simulink model "sistema_completo_discretizado_con_funciones"  (R2023b)
settings: Solver=VariableStepAuto  StartTime=0.0  StopTime=10.0  RelTol=1e-3
values from neighbouring files (symbols this model uses):
  alpha_Cu = 3.9e-3    (= 0.0039)    [controlador_foc_simulink.m]    (also in parametros_planta.m; params_subsistema_termico.m; sistema_completo_en_codigo.m)
  beq_nom = bm + bl_nom/r^2    (= 2.19444444444e-05)    [parametros_planta.m]    (also in params_subsistema_mecanico.m; sistema_completo_en_codigo.m)
  Cts = 0.818    [parametros_planta.m]    (also in params_subsistema_termico.m)
  Jeq_nom = Jm + Jl_nom/r^2    (= 1.97847222222e-05)    [params_subsistema_mecanico.m]    (also in sistema_completo_en_codigo.m)
  kg_eq_nom = g*kl_nom/r    (= 0.0204305208333)    [params_subsistema_mecanico.m]    (also in sistema_completo_en_codigo.m)
  L_d = 6.6e-3    (= 0.0066)    [controlador_foc_simulink.m]    (also in params_subsistema_electromagnetico.m; sistema_completo_en_codigo.m)
  L_l = 0.8e-3    (= 0.0008)    [controlador_foc_simulink.m]    (also in params_subsistema_electromagnetico.m; sistema_completo_en_codigo.m)
  L_q = 5.8e-3    (= 0.0058)    [controlador_foc_simulink.m]    (also in params_subsistema_electromagnetico.m; sistema_completo_en_codigo.m)
  lambda_m = 0.016    [controlador_foc_simulink.m]    (also in parametros_planta.m; params_subsistema_electromagnetico.m; sistema_completo_en_codigo.m)
  Pp = 3    [controlador_foc_simulink.m]    (also in parametros_planta.m; params_subsistema_electromagnetico.m; sistema_completo_en_codigo.m)
  r = 120.0    (= 120)    [controlador_foc_simulink.m]    (also in parametros_planta.m; params_subsistema_mecanico.m; sistema_completo_en_codigo.m)
  Rs_REF = 1.02    [controlador_foc_simulink.m]    (also in parametros_planta.m; params_subsistema_termico.m; sistema_completo_en_codigo.m)
  Rts_amb = 146.7    [parametros_planta.m]    (also in params_subsistema_termico.m)
  Tamb = Tamb_max    (= 40)    [parametros_planta.m]    (also in params_subsistema_termico.m; sistema_completo_en_codigo.m)
  Ts = interp_ts(Ts_ts,t)    [calcular_metricas_operacion.m]
  Ts_REF = 20.0    (= 20)    [controlador_foc_simulink.m]    (also in parametros_planta.m; params_subsistema_termico.m; sistema_completo_en_codigo.m)
undefined symbols (not defined in the file or in its folder): A_iabc, A_pos, A_T, A_v, B_iabc, B_pos, B_T, B_v, C_iabc, C_pos, C_T, C_v, D_iabc, D_pos, D_T, D_v
settings Model: Creator=Pc  LastModifiedBy=Pc

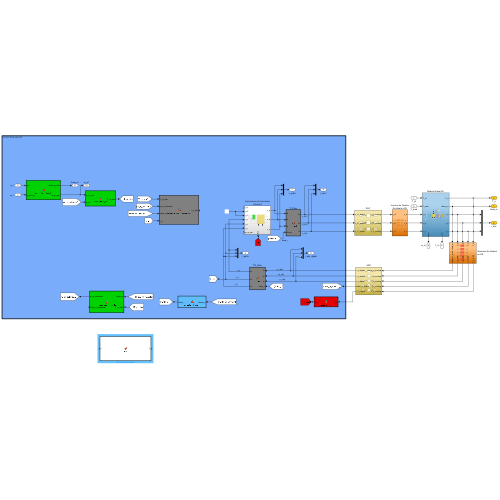
[thumbnail: Simulink's stored preview of the top-level diagram]
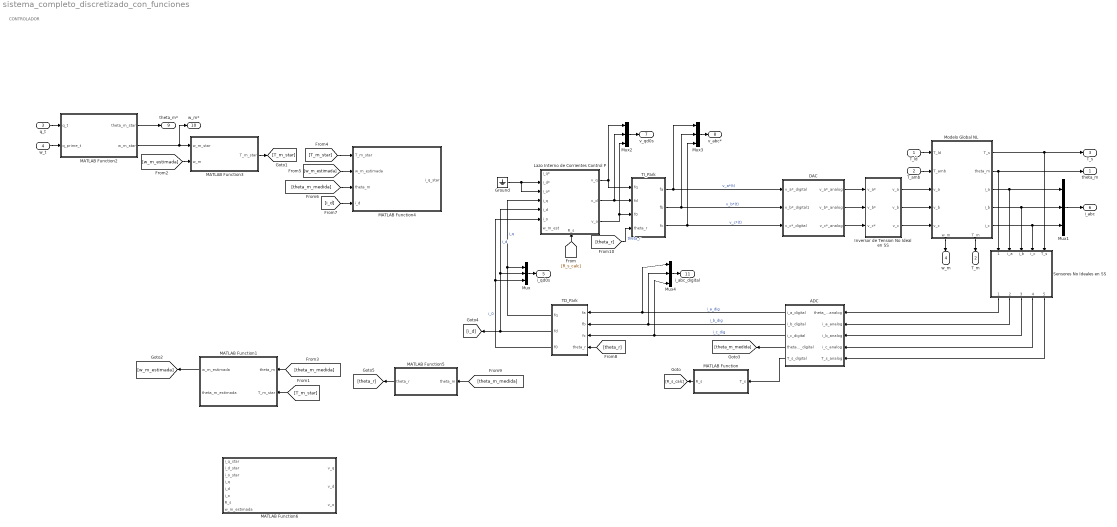
== system sistema_completo_discretizado_con_funciones ==
  note: CONTROLADOR
  T_ld : Inport
  T_amb : Inport  Port=2
  q_t : Inport  Port=3
  w_t : Inport  Port=4
  " ADC" : Subsystem
  DAC : Subsystem
  Ground : Ground
  Inversor de Tension No Ideal en SS : Subsystem
  Lazo Interno de Corrientes Control P : Subsystem
      settings: PortSchema="{\"entries\":[{\"content\":{\"sides\":[{\"content\":{\"connectorIds\":[\"In1\",\"In2\",\"In3\",\"In4\",\"In5\",\"In6\",\"In7\"]},\"type\":\"ConnectorPlacement.EquallySpacedRectSide\",\"uuid\":\"003130de-7086-42b2-88ab-1550be464119\"},{\"content\":{\"connectorIds\":[\"Out1\",\"Out2\",\"Out3\"],\"side\":\"RIGHT\"},\"type\":\"ConnectorPlacement.EquallySpacedRectSide\",\"uuid\":\"1ef26d10-ae91-4351-8dbc-50b579db1e66\"},{\"content\":{\"side\":\"TOP\"},\"type\":\"ConnectorPlacement.EquallySpacedRectSide\",\"uuid\":\"f8d5b360-b304-4c62-a3c0-e85b3671d199\"},{\"content\":{\"connectorIds\":[\"In8\"],\"side\":\"BOTTOM\"},\"type\":\"ConnectorPlacement.EquallySpacedRectSide\",\"uuid\":\"ca7bddea-434a-49b1-aeae-36f1f1b68346\"}]},\"type\":\"ConnectorPlacement.EquallySpacedConnector\",\"uuid\":\"97d0594b-d096-4b47-8675-ea576c5ffe32\"}],\"packageUris\":[\"http://schema.mathworks.com/mf0/Connector/R2020b\"],\"version\":\"1.0\"}"
  MATLAB Function : MATLAB Function  TreatAsAtomicUnit=on
  MATLAB Function1 : MATLAB Function  TreatAsAtomicUnit=on
  MATLAB Function2 : MATLAB Function  TreatAsAtomicUnit=on
  MATLAB Function3 : MATLAB Function  TreatAsAtomicUnit=on
  MATLAB Function4 : MATLAB Function  TreatAsAtomicUnit=on
  MATLAB Function5 : MATLAB Function  TreatAsAtomicUnit=on
  MATLAB Function6 : MATLAB Function  TreatAsAtomicUnit=on
  Modelo Global NL : Subsystem
      settings: PortSchema="{\"entries\":[{\"content\":{\"sides\":[{\"content\":{\"connectorIds\":[\"In1\",\"In2\",\"In3\",\"In4\",\"In5\"]},\"type\":\"ConnectorPlacement.EquallySpacedRectSide\",\"uuid\":\"386252be-5f39-4928-a151-52e681895a84\"},{\"content\":{\"connectorIds\":[\"Out1\",\"Out2\",\"Out3\",\"Out4\",\"Out5\"],\"side\":\"RIGHT\"},\"type\":\"ConnectorPlacement.EquallySpacedRectSide\",\"uuid\":\"aee83b90-e95b-4477-b157-a5534e7c5e6c\"},{\"content\":{\"side\":\"TOP\"},\"type\":\"ConnectorPlacement.EquallySpacedRectSide\",\"uuid\":\"e739b3f7-cae1-4498-b396-d13f7405e232\"},{\"content\":{\"connectorIds\":[\"Out6\",\"Out7\"],\"side\":\"BOTTOM\"},\"type\":\"ConnectorPlacement.EquallySpacedRectSide\",\"uuid\":\"86304fed-22cd-46a2-87e5-e7bae1c5cedf\"}]},\"type\":\"ConnectorPlacement.EquallySpacedConnector\",\"uuid\":\"c0eb110b-b212-4702-a1d5-9ec3ac2ff196\"}],\"packageUris\":[\"http://schema.mathworks.com/mf0/Connector/R2020b\"],\"version\":\"1.0\"}"
  Mux{,1..4} (5 alike) : Mux  Inputs=3
  Sensores No Ideales en SS : Subsystem
  TD_Park : MATLAB Function  TreatAsAtomicUnit=on
  TI_Park : MATLAB Function  TreatAsAtomicUnit=on
  theta_m : Outport
  T_m : Outport  Port=2
  T_s : Outport  Port=3
  w_m : Outport  Port=4
  i_qd0s : Outport  Port=5
  i_abc : Outport  Port=6
  v_qd0s : Outport  Port=7
  v_abc* : Outport  Port=8
  theta_m* : Outport  Port=9
  w_m* : Outport  Port=10
  i_abc_digital : Outport  Port=11
  wires:
  Sensores No Ideales en SS/5(T_s_med) -> " ADC"/5(T_s_analog)
  Modelo Global NL/6(w_m) -> w_m/1
  Modelo Global NL/5(i_c) -> Mux1/3, Sensores No Ideales en SS/4(i_c)
  TI_Park/3(fc) -> DAC/3(v_c*_digital), Mux3/3  "v_c*(t)"
  " ADC"/2(i_b_digital) -> Mux4/2, TD_Park/2(fb)  "i_b_dig"
  Modelo Global NL/4(i_b) -> Mux1/2, Sensores No Ideales en SS/3(i_b)
  Sensores No Ideales en SS/1(theta_m_med) -> " ADC"/1(theta_m_analog)
  T_amb/1 -> Modelo Global NL/2(T_amb)
  " ADC"/1(i_a_digital) -> Mux4/1, TD_Park/1(fa)  "i_a_dig"
  DAC/3(v_c*_analog) -> Inversor de Tension No Ideal en SS/3(v_c*)
  Modelo Global NL/1(T_s) -> Sensores No Ideales en SS/5(T_s), T_s/1
  Sensores No Ideales en SS/3(i_b_med) -> " ADC"/3(i_b_analog)
  MATLAB Function2/1(theta_m_star) -> theta_m*/1
  Mux/1 -> i_qd0s/1
  TD_Park/2(fd) -> [i_d], Lazo Interno de Corrientes Control P/5(i_d), Mux/2  "i_d"
  DAC/1(v_a*_analog) -> Inversor de Tension No Ideal en SS/1(v_a*)
  TI_Park/2(fb) -> DAC/2(v_b*_digital1), Mux3/2  "v_b*(t)"
  " ADC"/4(theta_m_digital) -> [theta_m_medida]
  Mux3/1 -> v_abc*/1
  [theta_r] -> TI_Park/4(theta_r)  "theta_r"
  DAC/2(v_b*_analog) -> Inversor de Tension No Ideal en SS/2(v_b*)
  Ground/1 -> Lazo Interno de Corrientes Control P/3(i_o*), Lazo Interno de Corrientes Control P/2(i_d*)
  TD_Park/3(f0) -> Mux/3, Lazo Interno de Corrientes Control P/6(i_o)  "i_0"
  MATLAB Function3/1(T_m_star) -> [T_m_star]
  TD_Park/1(fq) -> Mux/1, Lazo Interno de Corrientes Control P/4(i_q)  "i_q"
  Inversor de Tension No Ideal en SS/1(v_a) -> Modelo Global NL/3(v_a)
  Sensores No Ideales en SS/2(i_a_med) -> " ADC"/2(i_a_analog)
  Lazo Interno de Corrientes Control P/1(v_q) -> TI_Park/1(fq), Mux2/1
  MATLAB Function2/2(w_m_star) -> MATLAB Function3/1(w_m_star), w_m*/1
  MATLAB Function/1(R_s) -> [R_s_calc]
  Modelo Global NL/7(T_m) -> T_m/1
  " ADC"/5(T_s_digital) -> MATLAB Function/1(T_s)
  [R_s_calc] -> Lazo Interno de Corrientes Control P/8(R_s)
  Mux4/1 -> i_abc_digital/1
  Lazo Interno de Corrientes Control P/3(v_o) -> TI_Park/3(f0), Mux2/3
  Lazo Interno de Corrientes Control P/2(v_d) -> TI_Park/2(fd), Mux2/2
  Modelo Global NL/2(theta_m) -> theta_m/1, Sensores No Ideales en SS/1(theta_m)
  Mux2/1 -> v_qd0s/1
  Inversor de Tension No Ideal en SS/2(v_b) -> Modelo Global NL/4(v_b)
  Mux1/1 -> i_abc/1
  T_ld/1 -> Modelo Global NL/1(T_ld)
  TI_Park/1(fa) -> DAC/1(v_a*_digital), Mux3/1  "v_a*(t)"
  Inversor de Tension No Ideal en SS/3(v_c) -> Modelo Global NL/5(v_c)
  Modelo Global NL/3(i_a) -> Mux1/1, Sensores No Ideales en SS/2(i_a)
  Sensores No Ideales en SS/4(i_c_med) -> " ADC"/4(i_c_analog)
  " ADC"/3(i_c_digital) -> Mux4/3, TD_Park/3(fc)  "i_c_dig"
  MATLAB Function1/1(w_m_estimada) -> [w_m_estimada]
  [T_m_star] -> MATLAB Function1/2(T_m_star)
  q_t/1 -> MATLAB Function2/1(q_t)
  w_t/1 -> MATLAB Function2/2(q_prime_t)
  [w_m_estimada] -> MATLAB Function3/2(w_m)
  [T_m_star] -> MATLAB Function4/1(T_m_star)
  [w_m_estimada] -> MATLAB Function4/2(w_m_estimada)
  [theta_m_medida] -> MATLAB Function1/1(theta_m)
  [theta_m_medida] -> MATLAB Function4/3(theta_m)
  [i_d] -> MATLAB Function4/4(i_d)
  MATLAB Function5/1(theta_r) -> [theta_r]
  [theta_m_medida] -> MATLAB Function5/1(theta_m)
  [theta_r] -> TD_Park/4(theta_r)

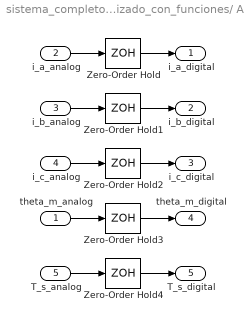
== system sistema_completo_discretizado_con_funciones/ ADC ==
  theta_m_analog : Inport
  i_a_analog : Inport  Port=2
  i_b_analog : Inport  Port=3
  i_c_analog : Inport  Port=4
  T_s_analog : Inport  Port=5
  Zero-Order Hold{,1..4} (5 alike) : ZeroOrderHold  SampleTime=Ts
  i_a_digital : Outport
  i_b_digital : Outport  Port=2
  i_c_digital : Outport  Port=3
  theta_m_digital : Outport  Port=4
  T_s_digital : Outport  Port=5
  wires:
  theta_m_analog/1 -> Zero-Order Hold3/1
  i_a_analog/1 -> Zero-Order Hold/1
  Zero-Order Hold/1 -> i_a_digital/1
  i_c_analog/1 -> Zero-Order Hold2/1
  i_b_analog/1 -> Zero-Order Hold1/1
  T_s_analog/1 -> Zero-Order Hold4/1
  Zero-Order Hold1/1 -> i_b_digital/1
  Zero-Order Hold2/1 -> i_c_digital/1
  Zero-Order Hold3/1 -> theta_m_digital/1
  Zero-Order Hold4/1 -> T_s_digital/1

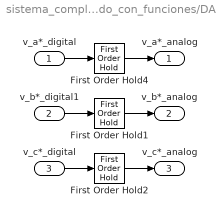
== system sistema_completo_discretizado_con_funciones/DAC ==
  v_a*_digital : Inport
  v_b*_digital1 : Inport  Port=2
  v_c*_digital : Inport  Port=3
  First Order Hold1 : FirstOrderHold  ErrorTolerance=inf  AllowContinuousInput=on
  First Order Hold2 : FirstOrderHold  ErrorTolerance=inf  AllowContinuousInput=on
  First Order Hold4 : FirstOrderHold  ErrorTolerance=inf  AllowContinuousInput=on
  v_a*_analog : Outport
  v_b*_analog : Outport  Port=2
  v_c*_analog : Outport  Port=3
  wires:
  v_c*_digital/1 -> First Order Hold2/1
  v_b*_digital1/1 -> First Order Hold1/1
  v_a*_digital/1 -> First Order Hold4/1
  First Order Hold4/1 -> v_a*_analog/1
  First Order Hold1/1 -> v_b*_analog/1
  First Order Hold2/1 -> v_c*_analog/1

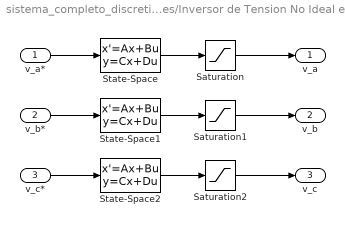
== system sistema_completo_discretizado_con_funciones/Inversor de Tension No Ideal en SS ==
  v_a* : Inport
  v_b* : Inport  Port=2
  v_c* : Inport  Port=3
  Saturation : Saturate  UpperLimit=39.19  LowerLimit=-39.19
  Saturation1 : Saturate  UpperLimit=39.19  LowerLimit=-39.19
  Saturation2 : Saturate  UpperLimit=39.19  LowerLimit=-39.19
  State-Space : StateSpace  A=A_v  B=B_v  C=C_v  D=D_v  InitialCondition=0
  State-Space1 : StateSpace  A=A_v  B=B_v  C=C_v  D=D_v  InitialCondition=0
  State-Space2 : StateSpace  A=A_v  B=B_v  C=C_v  D=D_v  InitialCondition=0
  v_a : Outport
  v_b : Outport  Port=2
  v_c : Outport  Port=3
  wires:
  Saturation1/1 -> v_b/1
  State-Space1/1 -> Saturation1/1
  Saturation/1 -> v_a/1
  v_c*/1 -> State-Space2/1
  Saturation2/1 -> v_c/1
  State-Space2/1 -> Saturation2/1
  v_b*/1 -> State-Space1/1
  State-Space/1 -> Saturation/1
  v_a*/1 -> State-Space/1

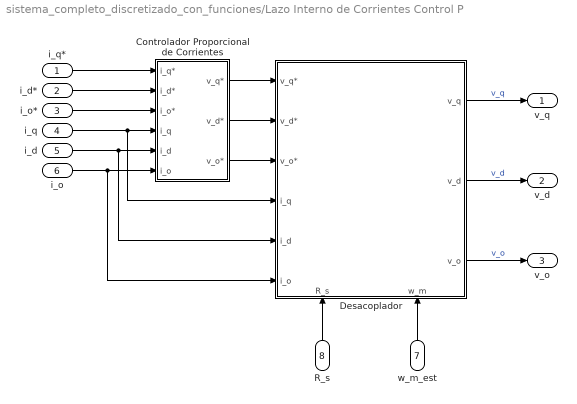
== system sistema_completo_discretizado_con_funciones/Lazo Interno de Corrientes Control P ==
  i_q* : Inport
  i_d* : Inport  Port=2
  i_o* : Inport  Port=3
  i_q : Inport  Port=4
  i_d : Inport  Port=5
  i_o : Inport  Port=6
  w_m_est : Inport  Port=7
  R_s : Inport  Port=8
  Controlador Proporcional de Corrientes : Subsystem
  Desacoplador : Subsystem
      settings: PortSchema="{\"entries\":[{\"content\":{\"sides\":[{\"content\":{\"connectorIds\":[\"In1\",\"In2\",\"In3\",\"In4\",\"In5\",\"In6\"]},\"type\":\"ConnectorPlacement.EquallySpacedRectSide\",\"uuid\":\"003130de-7086-42b2-88ab-1550be464119\"},{\"content\":{\"connectorIds\":[\"Out1\",\"Out2\",\"Out3\"],\"side\":\"RIGHT\"},\"type\":\"ConnectorPlacement.EquallySpacedRectSide\",\"uuid\":\"1ef26d10-ae91-4351-8dbc-50b579db1e66\"},{\"content\":{\"side\":\"TOP\"},\"type\":\"ConnectorPlacement.EquallySpacedRectSide\",\"uuid\":\"f8d5b360-b304-4c62-a3c0-e85b3671d199\"},{\"content\":{\"connectorIds\":[\"In7\",\"In8\"],\"side\":\"BOTTOM\"},\"type\":\"ConnectorPlacement.EquallySpacedRectSide\",\"uuid\":\"ed3aa2b2-0c88-4f8f-b202-0aa60a8551ab\"}]},\"type\":\"ConnectorPlacement.EquallySpacedConnector\",\"uuid\":\"97d0594b-d096-4b47-8675-ea576c5ffe32\"}],\"packageUris\":[\"http://schema.mathworks.com/mf0/Connector/R2020b\"],\"version\":\"1.0\"}"
  v_q : Outport
  v_d : Outport  Port=2
  v_o : Outport  Port=3
  wires:
  Desacoplador/3(v_o) -> v_o/1  "v_o"
  Controlador Proporcional de Corrientes/1(v_q*) -> Desacoplador/1(v_q*)
  Desacoplador/1(v_q) -> v_q/1  "v_q"
  w_m_est/1 -> Desacoplador/8(w_m)
  Controlador Proporcional de Corrientes/3(v_o*) -> Desacoplador/3(v_o*)
  i_d/1 -> Controlador Proporcional de Corrientes/5(i_d), Desacoplador/5(i_d)
  i_q/1 -> Controlador Proporcional de Corrientes/4(i_q), Desacoplador/4(i_q)
  i_o/1 -> Controlador Proporcional de Corrientes/6(i_o), Desacoplador/6(i_o)
  i_d*/1 -> Controlador Proporcional de Corrientes/2(i_d*)
  i_q*/1 -> Controlador Proporcional de Corrientes/1(i_q*)
  i_o*/1 -> Controlador Proporcional de Corrientes/3(i_o*)
  Controlador Proporcional de Corrientes/2(v_d*) -> Desacoplador/2(v_d*)
  R_s/1 -> Desacoplador/7(R_s)
  Desacoplador/2(v_d) -> v_d/1  "v_d"

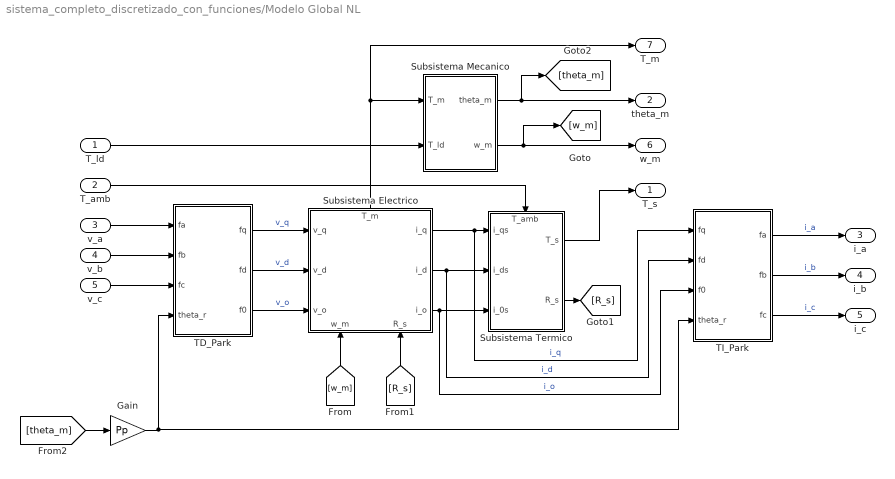
== system sistema_completo_discretizado_con_funciones/Modelo Global NL ==
  T_ld : Inport
  T_amb : Inport  Port=2
  v_a : Inport  Port=3
  v_b : Inport  Port=4
  v_c : Inport  Port=5
  Gain : Gain  Gain=Pp
  Subsistema Electrico : Subsystem
      settings: PortSchema="{\"entries\":[{\"content\":{\"sides\":[{\"content\":{\"connectorIds\":[\"In1\",\"In2\",\"In3\"]},\"type\":\"ConnectorPlacement.EquallySpacedRectSide\",\"uuid\":\"c7eb63ae-4015-4be9-a2f8-5ddbad38e871\"},{\"content\":{\"connectorIds\":[\"Out1\",\"Out2\",\"Out3\"],\"side\":\"RIGHT\"},\"type\":\"ConnectorPlacement.EquallySpacedRectSide\",\"uuid\":\"ed205027-9864-417a-9d2b-6eeb723ffec2\"},{\"content\":{\"connectorIds\":[\"Out4\"],\"side\":\"TOP\"},\"type\":\"ConnectorPlacement.EquallySpacedRectSide\",\"uuid\":\"5c5dee03-5728-4212-8fc2-a453d3484329\"},{\"content\":{\"connectorIds\":[\"In4\",\"In5\"],\"side\":\"BOTTOM\"},\"type\":\"ConnectorPlacement.EquallySpacedRectSide\",\"uuid\":\"494df340-b6d5-4f09-932e-9dbff39af1cf\"}]},\"type\":\"ConnectorPlacement.EquallySpacedConnector\",\"uuid\":\"0eeaea4c-3d80-4ebb-8c27-59b1b18764e9\"}],\"packageUris\":[\"http://schema.mathworks.com/mf0/Connector/R2020b\"],\"version\":\"1.0\"}"
  Subsistema Mecanico : Subsystem
  Subsistema Termico : Subsystem
      settings: PortSchema="{\"entries\":[{\"content\":{\"sides\":[{\"content\":{\"connectorIds\":[\"In1\",\"In2\",\"In3\"]},\"type\":\"ConnectorPlacement.EquallySpacedRectSide\",\"uuid\":\"5b1848a7-84bd-4673-a3fa-3976b4d0d5b9\"},{\"content\":{\"connectorIds\":[\"Out1\",\"Out2\"],\"side\":\"RIGHT\"},\"type\":\"ConnectorPlacement.EquallySpacedRectSide\",\"uuid\":\"feff3f8a-cd7c-43b1-91c3-7ab01b0b33a6\"},{\"content\":{\"connectorIds\":[\"In4\"],\"side\":\"TOP\"},\"type\":\"ConnectorPlacement.EquallySpacedRectSide\",\"uuid\":\"8de0b1b6-142f-442a-a92f-2baa615c6322\"}]},\"type\":\"ConnectorPlacement.EquallySpacedConnector\",\"uuid\":\"046fcb24-e0d9-4784-a784-7e36f9acbfbc\"}],\"packageUris\":[\"http://schema.mathworks.com/mf0/Connector/R2020b\"],\"version\":\"1.0\"}"
  TD_Park : MATLAB Function  TreatAsAtomicUnit=on
  TI_Park : MATLAB Function  TreatAsAtomicUnit=on
  T_s : Outport
  theta_m : Outport  Port=2
  i_a : Outport  Port=3
  i_b : Outport  Port=4
  i_c : Outport  Port=5
  w_m : Outport  Port=6
  T_m : Outport  Port=7
  wires:
  Subsistema Mecanico/1(theta_m) -> theta_m/1, [theta_m]
  TD_Park/2(fd) -> Subsistema Electrico/2(v_d)  "v_d"
  Subsistema Termico/1(T_s) -> T_s/1
  TD_Park/3(f0) -> Subsistema Electrico/3(v_o)  "v_o"
  Subsistema Mecanico/2(w_m) -> w_m/1, [w_m]
  [R_s] -> Subsistema Electrico/5(R_s)
  TI_Park/1(fa) -> i_a/1  "i_a"
  TD_Park/1(fq) -> Subsistema Electrico/1(v_q)  "v_q"
  Subsistema Electrico/4(T_m) -> T_m/1, Subsistema Mecanico/1(T_m)
  v_c/1 -> TD_Park/3(fc)
  Subsistema Electrico/2(i_d) -> Subsistema Termico/2(i_ds), TI_Park/2(fd)  "i_d"
  Subsistema Termico/2(R_s) -> [R_s]
  T_amb/1 -> Subsistema Termico/4(T_amb)
  T_ld/1 -> Subsistema Mecanico/2(T_ld)
  Subsistema Electrico/3(i_o) -> Subsistema Termico/3(i_0s), TI_Park/3(f0)  "i_o"
  TI_Park/2(fb) -> i_b/1  "i_b"
  Subsistema Electrico/1(i_q) -> TI_Park/1(fq), Subsistema Termico/1(i_qs)  "i_q"
  v_a/1 -> TD_Park/1(fa)
  v_b/1 -> TD_Park/2(fb)
  [w_m] -> Subsistema Electrico/4(w_m)
  TI_Park/3(fc) -> i_c/1  "i_c"
  [theta_m] -> Gain/1
  Gain/1 -> TD_Park/4(theta_r), TI_Park/4(theta_r)

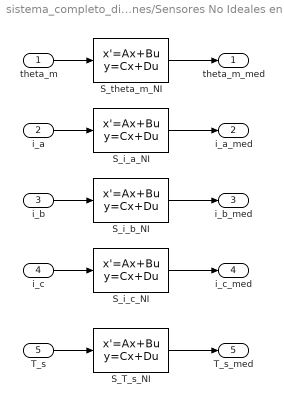
== system sistema_completo_discretizado_con_funciones/Sensores No Ideales en SS ==
  theta_m : Inport
  i_a : Inport  Port=2
  i_b : Inport  Port=3
  i_c : Inport  Port=4
  T_s : Inport  Port=5
  S_T_s_NI : StateSpace  A=A_T  B=B_T  C=C_T  D=D_T  InitialCondition=0
  S_i_a_NI : StateSpace  A=A_iabc  B=B_iabc  C=C_iabc  D=D_iabc  InitialCondition=0
  S_i_b_NI : StateSpace  A=A_iabc  B=B_iabc  C=C_iabc  D=D_iabc  InitialCondition=0
  S_i_c_NI : StateSpace  A=A_iabc  B=B_iabc  C=C_iabc  D=D_iabc  InitialCondition=0
  S_theta_m_NI : StateSpace  A=A_pos  B=B_pos  C=C_pos  D=D_pos  InitialCondition=0
  theta_m_med : Outport
  i_a_med : Outport  Port=2
  i_b_med : Outport  Port=3
  i_c_med : Outport  Port=4
  T_s_med : Outport  Port=5
  wires:
  S_i_b_NI/1 -> i_b_med/1
  i_b/1 -> S_i_b_NI/1
  T_s/1 -> S_T_s_NI/1
  i_c/1 -> S_i_c_NI/1
  S_i_c_NI/1 -> i_c_med/1
  S_T_s_NI/1 -> T_s_med/1
  i_a/1 -> S_i_a_NI/1
  S_theta_m_NI/1 -> theta_m_med/1
  theta_m/1 -> S_theta_m_NI/1
  S_i_a_NI/1 -> i_a_med/1

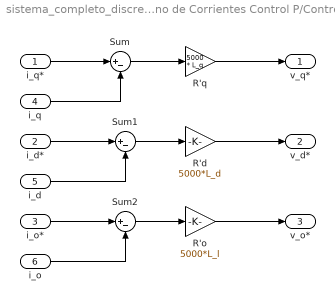
== system sistema_completo_discretizado_con_funciones/Lazo Interno de Corrientes Control P/Controlador Proporcional de Corrientes ==
  i_q* : Inport
  i_d* : Inport  Port=2
  i_o* : Inport  Port=3
  i_q : Inport  Port=4
  i_d : Inport  Port=5
  i_o : Inport  Port=6
  R'd : Gain  Gain=5000*L_d
  R'o : Gain  Gain=5000*L_l
  R'q : Gain  Gain=5000 * L_q
  Sum : Sum  Inputs=|+-
  Sum1 : Sum  Inputs=|+-
  Sum2 : Sum  Inputs=|+-
  v_q* : Outport
  v_d* : Outport  Port=2
  v_o* : Outport  Port=3
  wires:
  R'd/1 -> v_d*/1
  i_q/1 -> Sum/2
  i_d*/1 -> Sum1/1
  R'o/1 -> v_o*/1
  i_o*/1 -> Sum2/1
  Sum/1 -> R'q/1
  Sum1/1 -> R'd/1
  i_o/1 -> Sum2/2
  Sum2/1 -> R'o/1
  R'q/1 -> v_q*/1
  i_d/1 -> Sum1/2
  i_q*/1 -> Sum/1

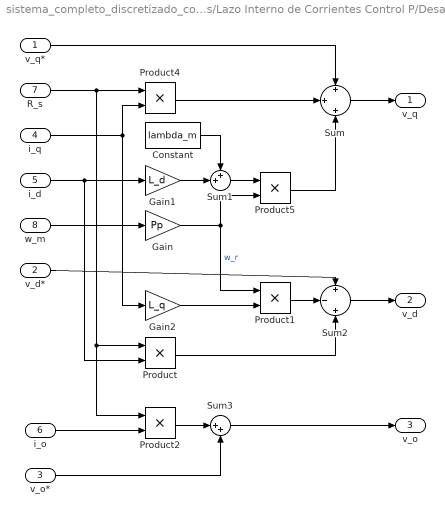
== system sistema_completo_discretizado_con_funciones/Lazo Interno de Corrientes Control P/Desacoplador ==
  v_q* : Inport
  v_d* : Inport  Port=2
  v_o* : Inport  Port=3
  i_q : Inport  Port=4
  i_d : Inport  Port=5
  i_o : Inport  Port=6
  R_s : Inport  Port=7
  w_m : Inport  Port=8
  Constant : Constant  Value=lambda_m
  Gain : Gain  Gain=Pp
  Gain1 : Gain  Gain=L_d
  Gain2 : Gain  Gain=L_q
  Product{,1..2,4..5} (5 alike) : Product
  Sum : Sum  Inputs=+|+|+
  Sum1 : Sum  Inputs=++|
  Sum2 : Sum  Inputs=+|-|+
  Sum3 : Sum  Inputs=|++
  v_q : Outport
  v_d : Outport  Port=2
  v_o : Outport  Port=3
  wires:
  R_s/1 -> Product/1, Product2/1, Product4/1
  Product2/1 -> Sum3/1
  v_d*/1 -> Sum2/1
  Gain/1 -> Product1/1, Product5/2  "w_r"
  Gain1/1 -> Sum1/2
  Product/1 -> Sum2/3
  Sum3/1 -> v_o/1
  i_d/1 -> Gain1/1, Product/2
  Product5/1 -> Sum/3
  Product1/1 -> Sum2/2
  Product4/1 -> Sum/2
  v_q*/1 -> Sum/1
  i_q/1 -> Gain2/1, Product4/2
  Sum/1 -> v_q/1
  i_o/1 -> Product2/2
  Sum1/1 -> Product5/1
  Sum2/1 -> v_d/1
  v_o*/1 -> Sum3/2
  w_m/1 -> Gain/1
  Constant/1 -> Sum1/1
  Gain2/1 -> Product1/2

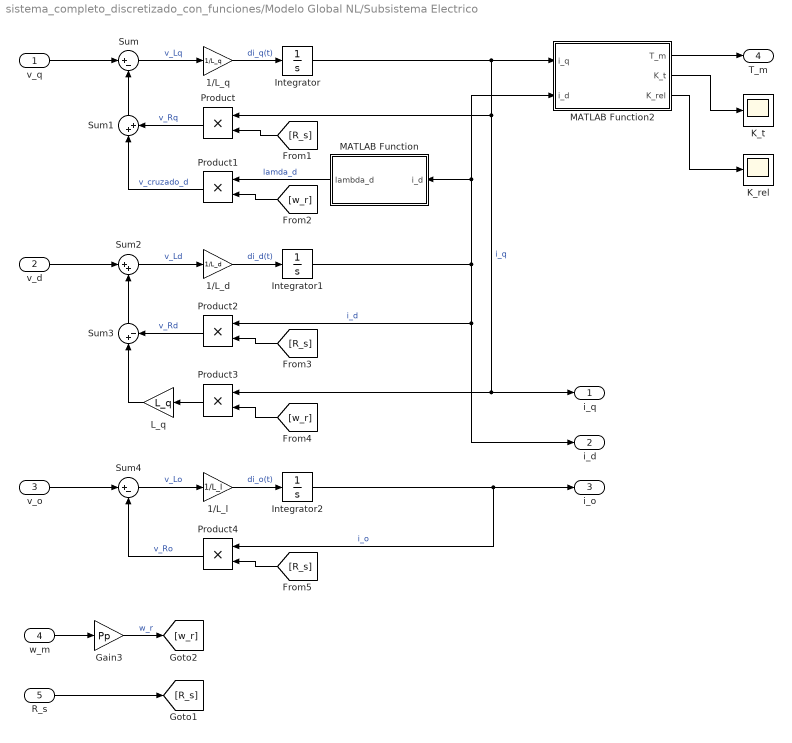
== system sistema_completo_discretizado_con_funciones/Modelo Global NL/Subsistema Electrico ==
  v_q : Inport
  v_d : Inport  Port=2
  v_o : Inport  Port=3
  w_m : Inport  Port=4
  R_s : Inport  Port=5
  1/L_d : Gain  Gain=1/L_d
  1/L_l : Gain  Gain=1/L_l
  1/L_q : Gain  Gain=1/L_q
  Gain3 : Gain  Gain=Pp
  Integrator : Integrator
  Integrator1 : Integrator
  Integrator2 : Integrator
  K_rel : Scope
  K_t : Scope
  L_q : Gain  Gain=L_q
  MATLAB Function : MATLAB Function  TreatAsAtomicUnit=on
  MATLAB Function2 : MATLAB Function  TreatAsAtomicUnit=on
  Product{,1..4} (5 alike) : Product
  Sum : Sum  Inputs=|+-
  Sum1 : Sum  Inputs=|++
  Sum2 : Sum  Inputs=|++
  Sum3 : Sum  Inputs=|+-
  Sum4 : Sum  Inputs=|+-
  i_q : Outport
  i_d : Outport  Port=2
  i_o : Outport  Port=3
  T_m : Outport  Port=4
  wires:
  Integrator/1 -> MATLAB Function2/1(i_q), Product/1, i_q/1, Product3/1  "i_q"
  Sum3/1 -> Sum2/2
  Product1/1 -> Sum1/1  "v_cruzado_d"
  Integrator1/1 -> MATLAB Function2/2(i_d), MATLAB Function/1(i_d), i_d/1, Product2/1  "i_d"
  Sum1/1 -> Sum/2
  1/L_d/1 -> Integrator1/1  "di_d(t)"
  MATLAB Function/1(lambda_d) -> Product1/1  "lamda_d"
  Sum4/1 -> 1/L_l/1  "v_Lo"
  [w_r] -> Product3/2
  Sum/1 -> 1/L_q/1  "v_Lq"
  1/L_l/1 -> Integrator2/1  "di_o(t)"
  Integrator2/1 -> i_o/1, Product4/1  "i_o"
  Product2/1 -> Sum3/2  "v_Rd"
  Product/1 -> Sum1/2  "v_Rq"
  [R_s] -> Product4/2
  Product3/1 -> L_q/1
  1/L_q/1 -> Integrator/1  "di_q(t)"
  Sum2/1 -> 1/L_d/1  "v_Ld"
  v_q/1 -> Sum/1
  [R_s] -> Product/2
  Product4/1 -> Sum4/2  "v_Ro"
  [w_r] -> Product1/2
  [R_s] -> Product2/2
  L_q/1 -> Sum3/1
  v_d/1 -> Sum2/1
  v_o/1 -> Sum4/1
  MATLAB Function2/1(T_m) -> T_m/1
  MATLAB Function2/3(K_rel) -> K_rel/1
  MATLAB Function2/2(K_t) -> K_t/1
  w_m/1 -> Gain3/1
  R_s/1 -> [R_s]
  Gain3/1 -> [w_r]  "w_r"

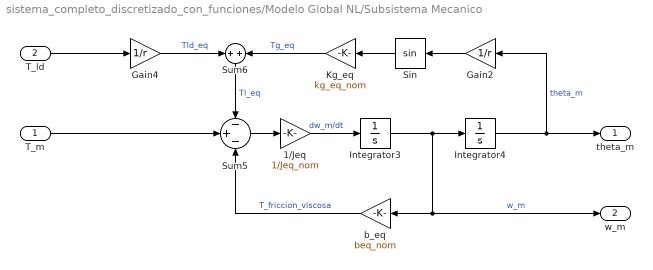
== system sistema_completo_discretizado_con_funciones/Modelo Global NL/Subsistema Mecanico ==
  T_m : Inport
  T_ld : Inport  Port=2
  1/Jeq : Gain  Gain=1/Jeq_nom
  Gain2 : Gain  Gain=1/r
  Gain4 : Gain  Gain=1/r
  Integrator3 : Integrator
  Integrator4 : Integrator
  Kg_eq : Gain  Gain=kg_eq_nom
  Sin : Trigonometry
  Sum5 : Sum  Inputs=-+-
  Sum6 : Sum  Inputs=+|+
  b_eq : Gain  Gain=beq_nom
  theta_m : Outport
  w_m : Outport  Port=2
  wires:
  Sin/1 -> Kg_eq/1
  Gain4/1 -> Sum6/1  "Tld_eq"
  Integrator4/1 -> theta_m/1, Gain2/1  "theta_m"
  Kg_eq/1 -> Sum6/2  "Tg_eq"
  Sum5/1 -> 1/Jeq/1
  b_eq/1 -> Sum5/3  "T_friccion_viscosa"
  T_m/1 -> Sum5/2
  Gain2/1 -> Sin/1
  Sum6/1 -> Sum5/1  "Tl_eq"
  Integrator3/1 -> w_m/1, b_eq/1, Integrator4/1  "w_m"
  T_ld/1 -> Gain4/1
  1/Jeq/1 -> Integrator3/1  "dw_m/dt"

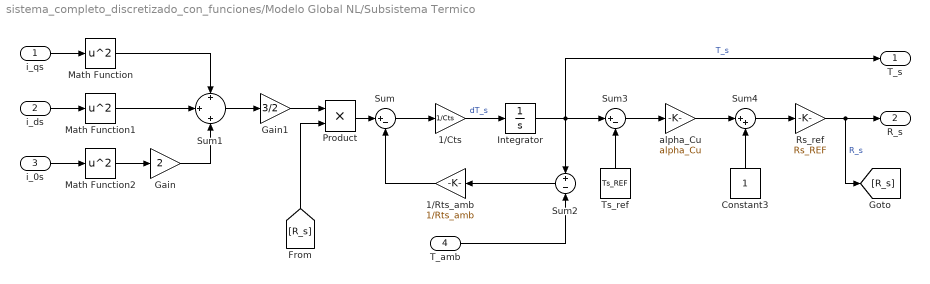
== system sistema_completo_discretizado_con_funciones/Modelo Global NL/Subsistema Termico ==
  i_qs : Inport
  i_ds : Inport  Port=2
  i_0s : Inport  Port=3
  T_amb : Inport  Port=4
  1/Cts : Gain  Gain=1/Cts
  1/Rts_amb : Gain  Gain=1/Rts_amb
  Constant3 : Constant
  Gain : Gain  Gain=2
  Gain1 : Gain  Gain=3/2
  Integrator : Integrator  InitialCondition=Tamb
  Math Function : Math  Operator=square
  Math Function1 : Math  Operator=square
  Math Function2 : Math  Operator=square
  Product : Product
  Rs_ref : Gain  Gain=Rs_REF
  Sum : Sum  Inputs=|+-
  Sum1 : Sum  Inputs=+|+|+
  Sum2 : Sum  Inputs=+-
  Sum3 : Sum  Inputs=|+-
  Sum4 : Sum  Inputs=|++
  Ts_ref : Constant  Value=Ts_REF
  alpha_Cu : Gain  Gain=alpha_Cu
  T_s : Outport
  R_s : Outport  Port=2
  wires:
  1/Cts/1 -> Integrator/1  "dT_s"
  Sum3/1 -> alpha_Cu/1
  Rs_ref/1 -> R_s/1, [R_s]  "R_s"
  Sum4/1 -> Rs_ref/1
  [R_s] -> Product/2
  i_ds/1 -> Math Function1/1
  Constant3/1 -> Sum4/2
  Integrator/1 -> T_s/1, Sum2/1, Sum3/1  "T_s"
  Math Function1/1 -> Sum1/2
  alpha_Cu/1 -> Sum4/1
  Sum2/1 -> 1/Rts_amb/1
  Product/1 -> Sum/1
  i_qs/1 -> Math Function/1
  Sum/1 -> 1/Cts/1
  T_amb/1 -> Sum2/2
  Math Function/1 -> Sum1/1
  i_0s/1 -> Math Function2/1
  1/Rts_amb/1 -> Sum/2
  Ts_ref/1 -> Sum3/2
  Math Function2/1 -> Gain/1
  Gain/1 -> Sum1/3
  Sum1/1 -> Gain1/1
  Gain1/1 -> Product/1

== matlab function sistema_completo_discretizado_con_funciones/MATLAB Function2 ==
  data: q_t input; theta_m_star output; q_prime_t input; w_m_star output
function [theta_m_star, w_m_star] = set_point_discreto(q_t, q_prime_t)
% SET_POINT_DISCRETO Genera las consignas de posición y velocidad 
% mecánicas referidas al eje del motor, a partir de comandos articulares.
% 
% Entradas:
%   q_t       : Consigna de posición articular [rad]
%   q_prime_t : Consigna de velocidad articular [rad/s]
%
% Salidas:
%   theta_m_star : Posición mecánica de referencia para el motor [rad]
%   w_m_star     : Velocidad mecánica de referencia para el motor [rad/s]
%
% Parámetros (Heredados del Workspace de MATLAB):
%   r   : Relación de transmisión del reductor planetario
%   T_s : Período de muestreo [s]

    % 1. Definición de variables de memoria (persistent)
    % Necesarias para recordar el pasado tanto en el derivador como en el integrador
    persistent q_t_prev q_prime_prev theta_int_prev

    % 2. Inicialización en el primer ciclo de ejecución (t=0)
    if isempty(q_t_prev)
        q_t_prev = q_t;             % Evita el pico (infinito) de la derivada en t=0
        q_prime_prev = q_prime_t;
        theta_int_prev = 0;         % El integrador arranca descargado
    end

    % 3. CÁLCULO NUMÉRICO DISCRETO
    
    % A. Derivador Discreto (Diferencia Hacia Atrás / Backward Euler)
    % Fórmula: dy[k] = (x[k] - x[k-1]) / Ts
    q_dot_derivado = (q_t - q_t_prev) / T_s;

    % B. Integrador Discreto (Método de Tustin / Trapezoidal)
    % Fórmula: y[k] = y[k-1] + (Ts/2) * (u[k] + u[k-1])
    theta_integrado = theta_int_prev + (T_s / 2) * (q_prime_t + q_prime_prev);

    % 4. SALIDAS DEL SISTEMA 
    % Aplicamos la relación de transmisión 'r' combinando las señales.
    % De este modo, la función responde sin importar qué entrada decida usar el usuario.
    theta_m_star = r * (q_t + theta_integrado);
    w_m_star     = r * (q_prime_t + q_dot_derivado);

    % 5. Actualización de memoria para el próximo ciclo
    q_t_prev = q_t;
    q_prime_prev = q_prime_t;
    theta_int_prev = theta_integrado;

end

== matlab function sistema_completo_discretizado_con_funciones/MATLAB Function3 ==
  data: w_m_star input; T_m_star output; w_m input
function T_m_star = controlador_pid(w_m_star, w_m)
% CONTROLADOR_PID Implementa el lazo de control cinemático discreto.
% Evita la derivación pura mediante memoria de estados y utiliza 
% aproximación trapezoidal (Tustin) para la acción integral.
%
% Entradas:
%   w_m_star : Velocidad mecánica de referencia [rad/s]
%   w_m      : Velocidad mecánica real/estimada [rad/s]
%
% Salida:
%   T_m_star : Consigna de torque electromagnético comandada [Nm]
%
% Parámetros (Heredados del Workspace de MATLAB):
%   Ksa_num  : Ganancia Proporcional (Kp)
%   Ksia_num : Ganancia Integral (Ki)
%   ba_num   : Ganancia Derivativa / Amortiguamiento Activo (Kd)
%   T_s      : Período de muestreo [s]
%   T_max    : Torque máximo permitido por el inversor [Nm] (Opcional para Anti-Windup)

    % 1. Definición de la memoria de los integradores (Variables de Estado)
    persistent I_estado e_prev

    % 2. Inicialización en el primer ciclo de ejecución (t=0)
    if isempty(I_estado)
        I_estado = 0;  % Integrador de la acción I arranca descargado
        e_prev = 0;    % Memoria del error para la acción derivativa
    end

    % 3. Cálculo del Error actual
    e_actual = w_m_star - w_m;

    % 4. ACCIÓN PROPORCIONAL
    P_action = Ksa_num * e_actual;

    % 5. ACCIÓN INTEGRAL (Método de Tustin / Trapezoidal)
    % Fórmula: y[k] = y[k-1] + (Ts/2) * Ki * (e[k] + e[k-1])
    I_action = I_estado + (T_s / 2) * Ksia_num * (e_actual + e_prev);

    % 6. ACCIÓN DERIVATIVA (Diferencia Hacia Atrás / Equivalente a Integrador en Cascada)
    % Se calcula usando la diferencia del error respecto al ciclo anterior.
    % Al dividir por T_s, digitalmente representa la pendiente sin necesidad
    % de un bloque derivador puro de Simulink que inestabilice el lazo.
    D_action = ba_num * (e_actual - e_prev) / T_s;

    % 7. CÁLCULO DE LA SALIDA TOTAL
    T_m_star_unbounded = P_action + I_action + D_action;

    % 8. SISTEMA ANTI-WINDUP Y SATURACIÓN DE SALIDA
    % Evita que el integrador matemático siga acumulando error (Windup)
    % si el sistema físico ha alcanzado el límite de torque del inversor.
    % Nota: T_max debe estar en el workspace (ej. 1.5 * Torque Nominal)
    T_max = 10; % Reemplazar por variable 'T_max' si se define en init_workspace.m
    
    if T_m_star_unbounded > T_max
        T_m_star = T_max;
        % Congelamos el integrador (No actualizamos I_estado)
    elseif T_m_star_unbounded < -T_max
        T_m_star = -T_max;
        % Congelamos el integrador (No actualizamos I_estado)
    else
        T_m_star = T_m_star_unbounded;
        % Zona lineal: Guardamos el valor integrado para el próximo ciclo
        I_estado = I_action; 
    end

    % 9. Actualización de la memoria de error para el próximo ciclo
    e_prev = e_actual;

end

== matlab function sistema_completo_discretizado_con_funciones/MATLAB Function4 ==
  data: T_m_star input; i_q_star output; w_m_estimada input; theta_m input; i_d input
function i_q_star = compensador_mecanico(T_m_star, w_m_estimada, theta_m, i_d)
% COMPENSADOR_MECANICO Calcula la corriente de referencia en el eje q (i_q*)
% aplicando Feedback Linearization para cancelar dinámicas mecánicas y
% mapear la consigna de torque a corriente.
%
% Entradas:
%   T_m_star     : Consigna de torque del controlador PID [Nm]
%   w_m_estimada : Velocidad mecánica estimada por el observador [rad/s]
%   theta_m      : Posición mecánica medida en el eje del motor [rad]
%   i_d          : Corriente medida/estimada en el eje d [A]
%
% Salida:
%   i_q_star     : Consigna de corriente para el eje de cuadratura [A]
%
% Parámetros (Heredados del Workspace de MATLAB):
%   b_eq  : Coeficiente de fricción viscosa equivalente [Nms/rad]
%   r     : Relación de transmisión del reductor planetario
%   K_g   : Constante de gravedad equivalente ((g * kl_nom) / r) [Nm]
%   K_t   : Constante de torque electromagnético nominal ((3/2)*Pp*lambda_m) [Nm/A]
%   K_rel : Constante de torque por reluctancia [Nm/A^2]

    % 1. Compensación Feedforward de Fricción Viscosa
    T_friccion = b_eq * w_m_estimada;

    % 2. Compensación Feedforward de Gravedad (Efecto pendular)
    % La posición del motor se divide por 'r' para proyectarla al ángulo real del brazo.
    T_gravedad = K_g * cos(theta_m / r);

    % 3. Torque Total Requerido
    % Se suma la orden del PID más las cancelaciones mecánicas.
    T_req = T_m_star + T_friccion + T_gravedad;

    % 4. Modulación de Torque a Corriente
    % La ecuación de torque es: T = (K_t + K_rel * i_d) * i_q
    % Despejamos i_q_star:
    Denominador_Torque = K_t + K_rel * i_d;

    % Proteccion de software industrial: Evitar división por cero
    % Si por algún error numérico el denominador es nulo, lo limitamos.
    if abs(Denominador_Torque) < 1e-6
        Denominador_Torque = sign(Denominador_Torque) * 1e-6;
        if Denominador_Torque == 0
            Denominador_Torque = 1e-6;
        end
    end

    % Cálculo final de la consigna de corriente
    i_q_star = T_req / Denominador_Torque;

end

== matlab function sistema_completo_discretizado_con_funciones/MATLAB Function5 ==
  data: theta_m input; theta_r output
function theta_r = calcular_theta_r(theta_m)
    theta_r = Pp * theta_m;
end

== matlab function sistema_completo_discretizado_con_funciones/MATLAB Function6 ==
  data: i_q_star input; v_q output; i_d_star input; i_o_star input; i_q input; i_d input; i_o input; R_s input; w_m_estimada input; v_d output; v_o output
function [v_q, v_d, v_o] = controlador_corriente(i_q_star, i_d_star, i_o_star, i_q, i_d, i_o, R_s, w_m_estimada)
% CONTROLADOR_CORRIENTE Lazo interno de corriente con desacoplamiento.
% Implementa el Control Proporcional (P) junto con la Linealización 
% por Realimentación Exacta para cancelar las no linealidades de la PMSM.
%
% Entradas:
%   i_q_star, i_d_star, i_o_star : Consignas de corriente (Referencias) [A]
%   i_q, i_d, i_o                : Corrientes reales medidas/transformadas [A]
%   R_s                          : Resistencia estatórica estimada actual [Ohms]
%   w_m_estimada                 : Velocidad mecánica estimada [rad/s]
%
% Salidas:
%   v_q, v_d, v_o : Tensiones de referencia para comandar al inversor [V]
%
% Parámetros (Heredados del Workspace de MATLAB):
%   R_q_prime : Ganancia proporcional del lazo q [Ohms]
%   R_d_prime : Ganancia proporcional del lazo d [Ohms]
%   R_o_prime : Ganancia proporcional del lazo homopolar 0 [Ohms]
%   L_q       : Inductancia del eje de cuadratura [H]
%   L_d       : Inductancia del eje directo [H]
%   Pp        : Número de pares de polos
%   lambda_m  : Flujo magnético de los imanes permanentes [Wb]

    % 1. CONTROLADOR PROPORCIONAL (Dinámica Deseada)
    % Cálculo del error de seguimiento
    e_q = i_q_star - i_q;
    e_d = i_d_star - i_d;
    e_o = i_o_star - i_o;
    
    % Generación de las tensiones auxiliares (v_bar)
    v_bar_q = R_q_prime * e_q;
    v_bar_d = R_d_prime * e_d;
    v_bar_o = R_o_prime * e_o;

    % 2. DESACOPLAMIENTO EXACTO (Feedback Linearization)
    % Sumamos a la tensión de control las dinámicas naturales de la 
    % planta para cancelarlas físicamente en el motor.

    % Eje en Cuadratura (q): Compensa caída óhmica y fuerza contraelectromotriz
    v_q = v_bar_q + R_s * i_q + Pp * w_m_estimada * (L_d * i_d + lambda_m);
    
    % Eje Directo (d): Compensa caída óhmica y acoplamiento por reluctancia cruzada
    v_d = v_bar_d + R_s * i_d - Pp * w_m_estimada * L_q * i_q;
    
    % Eje Homopolar (0): Compensa únicamente caída óhmica
    v_o = v_bar_o + R_s * i_o;

end

== matlab function sistema_completo_discretizado_con_funciones/Modelo Global NL/TD_Park ==
  data: fa input; fq output; fb input; fc input; theta_r input; fd output; f0 output
function [fq, fd, f0] = T_Park(fa, fb, fc, theta_r)
%#codegen
% Transformada directa de Park: abc -> qd0
% Convención usada:
% fq: eje q
% fd: eje d
% f0: componente homopolar

c1 = cos(theta_r);
c2 = cos(theta_r - 2*pi/3);
c3 = cos(theta_r + 2*pi/3);

s1 = sin(theta_r);
s2 = sin(theta_r - 2*pi/3);
s3 = sin(theta_r + 2*pi/3);

fq = (2/3)*(c1*fa + c2*fb + c3*fc);
fd = (2/3)*(s1*fa + s2*fb + s3*fc);
f0 = (1/3)*(fa + fb + fc);
end

== matlab function sistema_completo_discretizado_con_funciones/Modelo Global NL/Subsistema Electrico/MATLAB Function ==
  data: i_d input; lambda_d output; lambda_m parameter; L_d parameter
function lambda_d = calcular_flujo_d(i_d, lambda_m, L_d)
    % CALCULAR_FLUJO_D Calcula el flujo magnético total concatenado en el eje directo (d).
    %
    % Entradas:
    %   i_d      : Corriente instantánea en el eje d (Señal dinámica de entrada).
    %   lambda_m : Flujo de los imanes permanentes (Parámetro estático).
    %   L_d      : Inductancia del estator en el eje d (Parámetro estático).
    %
    % Salida:
    %   lambda_d : Flujo magnético total en el eje d.

    % Cálculo: Flujo de imanes + Flujo de reacción del inducido
    lambda_d = lambda_m + L_d * i_d;
end

== matlab function sistema_completo_discretizado_con_funciones/Modelo Global NL/Subsistema Electrico/MATLAB Function2 ==
  data: i_q input; i_d input; T_m output; Pp parameter; lambda_m parameter; L_d parameter; L_q parameter; K_t output; K_rel output
function [T_m, K_t, K_rel] = calcular_torque(i_q, i_d, Pp, lambda_m, L_d, L_q)
    % CALCULAR_TORQUE Calcula el torque electromagnético total de la máquina PMSM
    % y sus constantes equivalentes.
    % 
    % Entradas dinámicas (Inports):
    %   i_q      : Corriente en el eje en cuadratura [A].
    %   i_d      : Corriente en el eje directo [A].
    %
    % Parámetros estáticos (Parameters):
    %   P_p      : Número de pares de polos.
    %   lambda_m : Flujo magnético de los imanes permanentes [Wb].
    %   L_d      : Inductancia del eje d [H].
    %   L_q      : Inductancia del eje q [H].
    %
    % Salidas:
    %   T_m      : Torque electromagnético generado [N.m].
    %   K_t      : Constante de torque de alineación [N.m/A].
    %   K_rel    : Constante de torque de reluctancia [N.m/A^2].

    % 1. Cálculo de las constantes 
    K_t = (3/2) * Pp * lambda_m;
    K_rel = (3/2) * Pp * (L_d - L_q);

    % 2. Cálculo del torque electromagnético total
    T_m = K_t * i_q + K_rel * i_d * i_q;
end

== matlab function sistema_completo_discretizado_con_funciones/Modelo Global NL/TI_Park ==
  data: fq input; fa output; fd input; f0 input; theta_r input; fb output; fc output
function [fa, fb, fc] = TI_Park(fq, fd, f0, theta_r)
%#codegen
% Transformada inversa de Park: qd0 -> abc

fa = cos(theta_r)*fq ...
   + sin(theta_r)*fd ...
   + f0;

fb = cos(theta_r - 2*pi/3)*fq ...
   + sin(theta_r - 2*pi/3)*fd ...
   + f0;

fc = cos(theta_r + 2*pi/3)*fq ...
   + sin(theta_r + 2*pi/3)*fd ...
   + f0;
end

== matlab function sistema_completo_discretizado_con_funciones/TD_Park ==
  data: fa input; fq output; fb input; fc input; theta_r input; fd output; f0 output
function [fq, fd, f0] = T_Park(fa, fb, fc, theta_r)
%#codegen
% Transformada directa de Park: abc -> qd0
% Convención usada:
% fq: eje q
% fd: eje d
% f0: componente homopolar

c1 = cos(theta_r);
c2 = cos(theta_r - 2*pi/3);
c3 = cos(theta_r + 2*pi/3);

s1 = sin(theta_r);
s2 = sin(theta_r - 2*pi/3);
s3 = sin(theta_r + 2*pi/3);

fq = (2/3)*(c1*fa + c2*fb + c3*fc);
fd = (2/3)*(s1*fa + s2*fb + s3*fc);
f0 = (1/3)*(fa + fb + fc);
end

== matlab function sistema_completo_discretizado_con_funciones/TI_Park ==
  data: fq input; fa output; fd input; f0 input; theta_r input; fb output; fc output
function [fa, fb, fc] = TI_Park(fq, fd, f0, theta_r)
%#codegen
% Transformada inversa de Park: qd0 -> abc

fa = cos(theta_r)*fq ...
   + sin(theta_r)*fd ...
   + f0;

fb = cos(theta_r - 2*pi/3)*fq ...
   + sin(theta_r - 2*pi/3)*fd ...
   + f0;

fc = cos(theta_r + 2*pi/3)*fq ...
   + sin(theta_r + 2*pi/3)*fd ...
   + f0;
end

== matlab function sistema_completo_discretizado_con_funciones/MATLAB Function ==
  data: T_s input; R_s output
function R_s = estimar_Rs(T_s)
% ESTIMAR_RS Calcula la resistencia del bobinado del estator
% compensando la no linealidad térmica producida por efecto Joule.
%
% Entradas:
%   T_s     : Temperatura actual digitalizada del estator [°C] 
%
% Parámetros (Heredados del Workspace de MATLAB):
%   RsREF   : Resistencia nominal del motor [Ohms] 
%   alphaCu : Coeficiente de temperatura del cobre [1/°C] 
%   T_sREF  : Temperatura de referencia [°C] 
%
% Salida:
%   R_s     : Resistencia operativa estimada [Ohms] 

    % 1. Saturación de seguridad para la lectura del sensor
    % (Evita inestabilidad del controlador si el ADC lee ruido extremo 
    % o si el termopar se desconecta).
    if T_s < -20
        T_s_segura = -20;
    elseif T_s > 150
        T_s_segura = 150; % Temperatura máxima de la clase de aislamiento
    else
        T_s_segura = T_s;
    end

    % 2. Cálculo del incremento de temperatura
    Delta_T = T_s_segura - T_sREF;

    % 3. Aplicación de la Ecuación (13) del modelo físico
    R_s = RsREF * (1 + alphaCu * Delta_T);
    
end

== matlab function sistema_completo_discretizado_con_funciones/MATLAB Function1 ==
  data: theta_m input; T_m_star input; w_m_estimada output; theta_m_estimada output
function [w_m_estimada, theta_m_estimada] = observador_estado(theta_m, T_m_star)
% OBSERVADOR_ESTADO Implementación en código del Observador de Estado 
% Reducido Extendido utilizando integración discreta de Tustin.
%
% Entradas:
%   T_m_star : Consigna de torque electromagnético [Nm]
%   theta_m  : Posición mecánica real medida por el encoder [rad]
%
% Salidas:
%   w_m_estimada     : Velocidad mecánica estimada [rad/s]
%   theta_m_estimada : Posición mecánica estimada [rad]
%
% Parámetros (Heredados del Workspace de MATLAB):
%   Jeq                : Inercia equivalente del sistema [kg*m^2]
%   K_eth_ext_agresivo : Ganancia L1 del observador (Posición)
%   K_ew_ext_agresivo  : Ganancia L2 del observador (Velocidad)
%   K_ei_ext_agresivo  : Ganancia L3 del observador (Estado Extendido/Perturbación)
%   T_s                : Período de muestreo [s]

    % 1. Definición de la memoria del integrador (Variables de Estado)
    % Las variables 'persistent' mantienen su valor entre cada ejecución del bloque.
    persistent th_est w_est Tld_est
    persistent d_th_prev d_w_prev d_Tld_prev

    % 2. Inicialización (Se ejecuta solo en t=0)
    if isempty(th_est)
        th_est = 0;   % Condición inicial de posición estimada
        w_est = 0;    % Condición inicial de velocidad estimada
        Tld_est = 0;  % Condición inicial de torque de perturbación estimado
        
        d_th_prev = 0;
        d_w_prev = 0;
        d_Tld_prev = 0;
    end

    % 3. Asignación de las Salidas Actuales
    % Entregamos los estados calculados en el ciclo anterior.
    theta_m_estimada = th_est;
    w_m_estimada = w_est;

    % 4. Dinámica del Observador (Ecuaciones Diferenciales)
    % Cálculo del error de estimación
    e_theta = theta_m - theta_m_estimada;
    
    % Cálculo de las derivadas actuales (x_dot = A*x + B*u + L*e)
    % Nota: El estado extendido Tld_est agrupa fricción y carga externa.
    d_th_actual  = w_m_estimada + K_eth_ext_agresivo * e_theta;
    d_w_actual   = (1 / Jeq) * (T_m_star - Tld_est) + K_ew_ext_agresivo * e_theta;
    d_Tld_actual = K_ei_ext_agresivo * e_theta;

    % 5. Integración Discreta Numérica (Método Trapezoidal / Tustin)
    % Fórmula: y[k+1] = y[k] + (Ts/2) * (dy[k] + dy[k-1])
    % Actualizamos las variables persistentes para el PRÓXIMO ciclo.
    th_est  = th_est  + (T_s / 2) * (d_th_actual  + d_th_prev);
    w_est   = w_est   + (T_s / 2) * (d_w_actual   + d_w_prev);
    Tld_est = Tld_est + (T_s / 2) * (d_Tld_actual + d_Tld_prev);

    % 6. Actualización de la memoria de derivadas para el próximo ciclo
    d_th_prev  = d_th_actual;
    d_w_prev   = d_w_actual;
    d_Tld_prev = d_Tld_actual;
    
end
